simulink model "s360159_sim_MPC"  (R2025b)
settings: Solver=VariableStepAuto  StartTime=0.0  StopTime=t_sim  RelTol=1e-3
values from neighbouring files (symbols this model uses):
  C = zpk(tf(S,R,Ts))    [s360159_design.m]    (also in s360159_design_MPC.m = [1 0])
  md = MPCInit(Ad,Bd,Cy,Cz,Dz,Cc,Dc,Hp,Hw,zblk,Hu,ublk,du_max,du_min,u_max,u_min,z_max,z_min,Q,R,[],[],Ts,0,'qp_as')    [s360159_design_MPC.m]
  r = 1    [s360159_design_MPC.m]
libraries: cstblocks x1
settings Model: Creator=giovannimasi  LastModifiedBy=giovannimasi

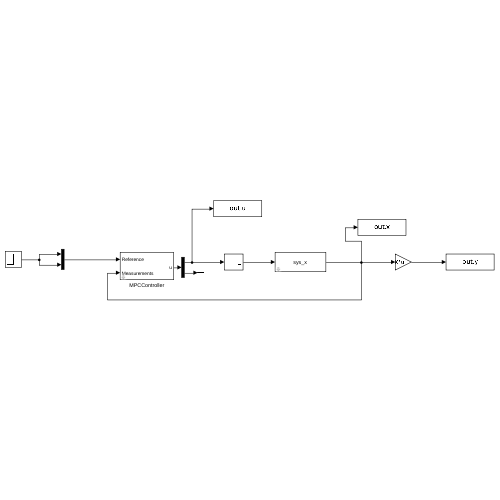
[thumbnail: Simulink's stored preview of the top-level diagram]
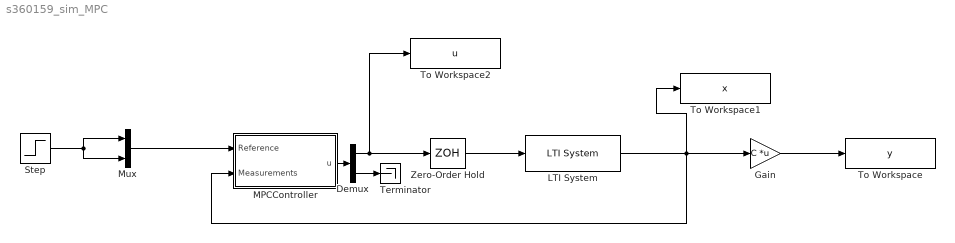
== system s360159_sim_MPC ==
  Demux : Demux  Outputs=2
  Gain : Gain  Gain=C  Multiplication=Matrix(K*u)
  LTI System : cstblocks/LTI System  sys=sys_x  IC=x0  PadeOrder=0
  MPCController : Subsystem  mask{md=md}
      mask prompts: md "MPCData"
  Mux : Mux  Inputs=2
  Step : Step  Time=0  After=r  SampleTime=0
  Terminator : Terminator
  To Workspace : ToWorkspace  VariableName=y  SaveFormat=Timeseries  SampleTime=-1
  To Workspace1 : ToWorkspace  VariableName=x  SaveFormat=Timeseries  SampleTime=-1
  To Workspace2 : ToWorkspace  VariableName=u  SaveFormat=Timeseries  SampleTime=-1
  Zero-Order Hold : ZeroOrderHold  SampleTime=-1
  wires:
  LTI System/1 -> To Workspace1/1, Gain/1, MPCController/2(Measurements)
  Gain/1 -> To Workspace/1
  Zero-Order Hold/1 -> LTI System/1
  MPCController/1(u) -> Demux/1
  Demux/1 -> To Workspace2/1, Zero-Order Hold/1
  Demux/2 -> Terminator/1
  Mux/1 -> MPCController/1(Reference)
  Step/1 -> Mux/2, Mux/1

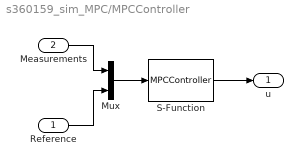
== system s360159_sim_MPC/MPCController ==
  Reference : Inport
  Measurements : Inport  Port=2
  Mux : Mux  Inputs=2
  S-Function : S-Function  FunctionName=MPCController  Parameters=md  SFunctionDeploymentMode=off  EnableBusSupport=off
  u : Outport
  wires:
  Mux/1 -> S-Function/1
  Measurements/1 -> Mux/1
  Reference/1 -> Mux/2
  S-Function/1 -> u/1
